simulink model "Impedence_rrbot"  (R2021a)
settings: Solver=FixedStepAuto  StartTime=0.0  StopTime=inf  RelTol=1e-3
model workspace (MAT data in the model file):
  SL_ROS_VariableLengthArrays_MaxSizes.CommonInfo.ArrayTruncateAction = 'EmitWarning'
  SL_ROS_VariableLengthArrays_MaxSizes.MsgTypeMap = containers.Map
  SL_ROS_VariableLengthArrays_MaxSizes.MsgTypeMap.serialization.keys = {'sensor_msgs/JointState'}
  SL_ROS_VariableLengthArrays_MaxSizes.MsgTypeMap.serialization.values{1}(1).PropertyName = 'Effort'
  SL_ROS_VariableLengthArrays_MaxSizes.MsgTypeMap.serialization.values{1}(1).DataType = 'double'
  SL_ROS_VariableLengthArrays_MaxSizes.MsgTypeMap.serialization.values{1}(1).MaxLength = 3
  SL_ROS_VariableLengthArrays_MaxSizes.MsgTypeMap.serialization.values{1}(2).PropertyName = 'Name'
  SL_ROS_VariableLengthArrays_MaxSizes.MsgTypeMap.serialization.values{1}(2).DataType = 'std_msgs/String'
  SL_ROS_VariableLengthArrays_MaxSizes.MsgTypeMap.serialization.values{1}(2).MaxLength = 16
  SL_ROS_VariableLengthArrays_MaxSizes.MsgTypeMap.serialization.values{1}(3).PropertyName = 'Position'
  SL_ROS_VariableLengthArrays_MaxSizes.MsgTypeMap.serialization.values{1}(3).DataType = 'double'
  SL_ROS_VariableLengthArrays_MaxSizes.MsgTypeMap.serialization.values{1}(3).MaxLength = 3
  SL_ROS_VariableLengthArrays_MaxSizes.MsgTypeMap.serialization.values{1}(4).PropertyName = 'Velocity'
  SL_ROS_VariableLengthArrays_MaxSizes.MsgTypeMap.serialization.values{1}(4).DataType = 'double'
  SL_ROS_VariableLengthArrays_MaxSizes.MsgTypeMap.serialization.values{1}(4).MaxLength = 3
  SL_ROS_VariableLengthArrays_MaxSizes.MsgTypeMap.serialization.uniformity = 0
  SL_ROS_VariableLengthArrays_MaxSizes.MsgTypeMap.serialization.keyType = 'char'
  SL_ROS_VariableLengthArrays_MaxSizes.MsgTypeMap.serialization.valueType = 'any'
undefined symbols (not defined in the file): B_imp, G, K_imp, M, V1
libraries: robotlib x7
settings Model: Creator=reaperj  LastModifiedBy=reaperj
settings OptimizationCC: EnhancedBackFolding=on  PassReuseOutputArgsAs=Individual arguments  ZeroExternalMemoryAtStartup=off  ZeroInternalMemoryAtStartup=off  MaxStackSize=64  OptimizeBlockOrder=speed  DifferentSizesBufferReuse=on  OptimizationCustomize=off  EfficientTunableParamExpr=on
settings DebuggingCC: ParameterTunabilityLossMsg=error
settings HardwareCC: ProdBitPerPointer=32  ProdBitPerSizeT=32  ProdBitPerPtrDiffT=32  ProdLargestAtomicFloat=None  ProdIntDivRoundTo=Undefined  ProdEndianess=Unspecified  ProdWordSize=32  ProdHWDeviceType=Generic->Unspecified (assume 32-bit Generic)  UseEmbeddedCoderFeatures=off
settings SFSimCC: MATLABDynamicMemAlloc=off
settings RTWCC: SystemTargetFile=ert.tlc  HardwareBoard=Robot Operating System (ROS)  TLCOptions="-aInlineSetEventsForThisBaseRateFcn=TLC_FALSE -aSuppressMultiTaskScheduler=TLC_FALSE  -aRateBasedStepFcn=0"  TemplateMakefile=ert_default_tmf  Toolchain=Catkin  TargetLang=C++
settings CodeAppCC: ForceParamTrailComments=on  IgnoreCustomStorageClasses=off  OperatorAnnotations=on  SimulinkDataObjDesc=on  SFDataObjDesc=on  InsertBlockDesc=on
settings ERTTargetCC: SupportNonInlinedSFcns=on

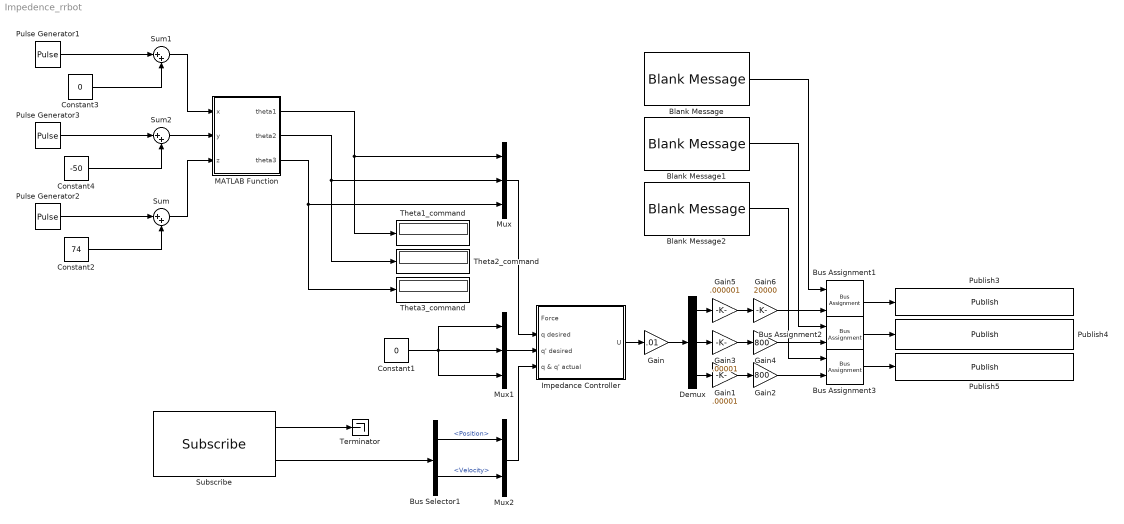
== system Impedence_rrbot ==
  Blank Message : robotlib/Blank Message  messageClass=Message  entityType=std_msgs/Float64  messageType=std_msgs/Float64  SampleTime=-1  legacyBusStruct=off
  Blank Message1 : robotlib/Blank Message  messageClass=Message  entityType=std_msgs/Float64  messageType=std_msgs/Float64  SampleTime=-1  legacyBusStruct=off
  Blank Message2 : robotlib/Blank Message  messageClass=Message  entityType=std_msgs/Float64  messageType=std_msgs/Float64  SampleTime=-1  legacyBusStruct=off
  Bus Assignment1 : BusAssignment  AssignedSignals=Data
  Bus Assignment2 : BusAssignment  AssignedSignals=Data
  Bus Assignment3 : BusAssignment  AssignedSignals=Data
  Bus Selector1 : BusSelector  OutputSignals=Position,Velocity
  Constant1 : Constant  Value=0
  Constant2 : Constant  Value=74
  Constant3 : Constant  Value=0
  Constant4 : Constant  Value=-50
  Demux : Demux  Outputs=3
  Gain : Gain  Gain=.01
  Gain1 : Gain  Gain=.00001
  Gain2 : Gain  Gain=800
  Gain3 : Gain  Gain=.00001
  Gain4 : Gain  Gain=800
  Gain5 : Gain  Gain=.000001
  Gain6 : Gain  Gain=20000
  Impedance Controller : Subsystem
  MATLAB Function : MATLAB Function  TreatAsAtomicUnit=on
  Mux : Mux  Inputs=3
  Mux1 : Mux  Inputs=3
  Mux2 : Mux  Inputs=2
  Publish3 : robotlib/Publish  topicSource=Select from ROS network  topic=/iiwa/joint1_effort_controller/command  messageType=std_msgs/Float64  legacyBusStruct=off  messageQueueLength=1
  Publish4 : robotlib/Publish  topicSource=Select from ROS network  topic=/iiwa/joint2_effort_controller/command  messageType=std_msgs/Float64  legacyBusStruct=off  messageQueueLength=1
  Publish5 : robotlib/Publish  topicSource=Select from ROS network  topic=/iiwa/joint4_effort_controller/command  messageType=std_msgs/Float64  legacyBusStruct=off  messageQueueLength=1
  Pulse Generator1 : DiscretePulseGenerator  PulseType=Time based  Amplitude=0  Period=300  PulseWidth=50
  Pulse Generator2 : DiscretePulseGenerator  PulseType=Time based  Amplitude=0  Period=300  PulseWidth=50  PhaseDelay=150
  Pulse Generator3 : DiscretePulseGenerator  PulseType=Time based  Amplitude=0  Period=300  PulseWidth=50  PhaseDelay=150
  Subscribe : robotlib/Subscribe  topicSource=Select from ROS network  topic=/iiwa/joint_states  messageType=sensor_msgs/JointState  SampleTime=.1  legacyBusStruct=off  messageQueueLength=1
  Sum : Sum  Inputs=|++
  Sum1 : Sum  Inputs=|++
  Sum2 : Sum  Inputs=|++
  Terminator : Terminator
  Theta1_command : Display
  Theta2_command : Display
  Theta3_command : Display
  wires:
  Bus Assignment2/1 -> Publish4/1
  Bus Assignment3/1 -> Publish5/1
  Blank Message2/1 -> Bus Assignment3/1
  Bus Assignment1/1 -> Publish3/1
  Blank Message/1 -> Bus Assignment1/1
  Impedance Controller/1(U) -> Gain/1
  MATLAB Function/3(theta3) -> Theta3_command/1, Mux/3
  Sum1/1 -> MATLAB Function/1(x)
  MATLAB Function/2(theta2) -> Theta2_command/1, Mux/2
  MATLAB Function/1(theta1) -> Theta1_command/1, Mux/1
  Mux/1 -> Impedance Controller/2(q desired)
  Mux1/1 -> Impedance Controller/3(q' desired)
  Subscribe/1 -> Terminator/1
  Bus Selector1/1 -> Mux2/1  "<Position>"
  Subscribe/2 -> Bus Selector1/1
  Bus Selector1/2 -> Mux2/2  "<Velocity>"
  Mux2/1 -> Impedance Controller/4(q & q' actual)
  Gain/1 -> Demux/1
  Constant1/1 -> Mux1/3, Mux1/1, Mux1/2
  Demux/3 -> Gain1/1
  Gain6/1 -> Bus Assignment1/2
  Gain1/1 -> Gain2/1
  Demux/1 -> Gain5/1
  Demux/2 -> Gain3/1
  Gain3/1 -> Gain4/1
  Gain5/1 -> Gain6/1
  Blank Message1/1 -> Bus Assignment2/1
  Sum/1 -> MATLAB Function/3(z)
  Gain2/1 -> Bus Assignment3/2
  Gain4/1 -> Bus Assignment2/2
  Pulse Generator2/1 -> Sum/1
  Constant2/1 -> Sum/2
  Pulse Generator1/1 -> Sum1/1
  Constant3/1 -> Sum1/2
  Constant4/1 -> Sum2/2
  Pulse Generator3/1 -> Sum2/1
  Sum2/1 -> MATLAB Function/2(y)

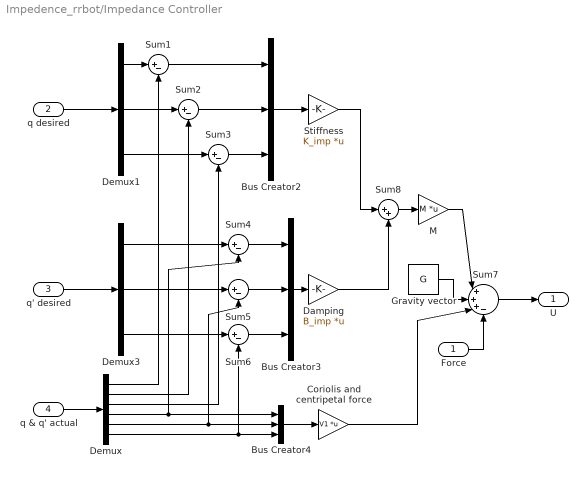
== system Impedence_rrbot/Impedance Controller ==
  Force : Inport
  q desired : Inport  Port=2
  q' desired : Inport  Port=3
  q & q' actual : Inport  Port=4
  Bus Creator2 : BusCreator  Inputs=3
  Bus Creator3 : BusCreator  Inputs=3
  Bus Creator4 : BusCreator  Inputs=3
  Coriolis and centripetal force : Gain  Gain=V1  Multiplication=Matrix(K*u)
  Damping : Gain  Gain=B_imp  Multiplication=Matrix(K*u)
  Demux : Demux  Outputs=6
  Demux1 : Demux  Outputs=3
  Demux3 : Demux  Outputs=3
  Gravity vector : Constant  Value=G  VectorParams1D=off
  M : Gain  Gain=M  Multiplication=Matrix(K*u)
  Stiffness : Gain  Gain=K_imp  Multiplication=Matrix(K*u)
  Sum{1..6} (6 alike) : Sum  Inputs=|+-
  Sum7 : Sum  Inputs=|+++-
  Sum8 : Sum  Inputs=|++
  U : Outport
  wires:
  Sum8/1 -> M/1
  Sum6/1 -> Bus Creator3/3
  Stiffness/1 -> Sum8/1
  Demux/3 -> Sum3/2
  Sum1/1 -> Bus Creator2/1
  Force/1 -> Sum7/4
  Bus Creator4/1 -> Coriolis and centripetal force/1
  Bus Creator2/1 -> Stiffness/1
  Demux/5 -> Bus Creator4/2, Sum5/2
  Sum5/1 -> Bus Creator3/2
  Demux/4 -> Bus Creator4/1, Sum4/2
  Demux/6 -> Bus Creator4/3, Sum6/2
  Sum2/1 -> Bus Creator2/2
  Demux/1 -> Sum1/2
  Bus Creator3/1 -> Damping/1
  Sum4/1 -> Bus Creator3/1
  Demux3/1 -> Sum4/1
  Sum3/1 -> Bus Creator2/3
  Demux/2 -> Sum2/2
  M/1 -> Sum7/1
  Damping/1 -> Sum8/2
  Demux3/3 -> Sum6/1
  q & q' actual/1 -> Demux/1
  Sum7/1 -> U/1
  Demux1/3 -> Sum3/1
  Demux1/1 -> Sum1/1
  Demux1/2 -> Sum2/1
  Demux3/2 -> Sum5/1
  Gravity vector/1 -> Sum7/2
  Coriolis and centripetal force/1 -> Sum7/3
  q desired/1 -> Demux1/1
  q' desired/1 -> Demux3/1

== matlab function Impedence_rrbot/MATLAB Function ==
  data: x input; theta1 output; y input; z input; theta2 output; theta3 output
%% Inverse Kinematics
function [theta1, theta2, theta3] = invk(x,y,z)

a1 = 34; a2 = 40; a3 = 52.6;
%a1 = 160 ;a2 = 100 ; a3 = 50;
r1 = sqrt(x^2 + y^2);
r2 = a1 - z;
if(r1== 0 && r2>=0)
    phi2 = pi/2;
elseif(r1== 0 && r2<0)
    phi2 = -pi/2;
else
    phi2 = atan(r2/r1);
end

r3 = sqrt(r1^2 + r2^2);
if(r3== 0)
    phi1 = 0;
else
    phi1 = acos((a3^2 - a2^2 - r3^2)/(-2*a2*r3));
end

phi3 = acos((r3^2 - a2^2 - a3^2)/(-2*a2*a3));

if(y == 0)
    theta1 = 0 ;
else
    theta1 = atan(y/x);
end

theta2 = phi2 - phi1 ;
theta3 = - pi + phi3;

theta1 = theta1 + (pi/2) ;
theta2 = theta2 + (pi/2);


end
